simulink model "SwcCanSendFaultV2"  (R2021b)
settings: Solver=ode1  StartTime=0.0  StopTime=15  FixedStep=0.01  RelTol=1e-3
PostLoadFcn:
  | CCM_Parameter
values from neighbouring files (symbols this model uses):
  Fault0x01 = FaultCodeGen(1,timeserise0x01)    [FaultCodeGenerate.m]
  Fault0x02 = FaultCodeGen(2,timeserise0x02)    [FaultCodeGenerate.m]
  Fault0x03 = FaultCodeGen(3,timeserise0x03)    [FaultCodeGenerate.m]
  Fault0x04 = FaultCodeGen(4,timeserise0x04)    [FaultCodeGenerate.m]
  Fault0x05 = FaultCodeGen(5,timeserise0x05)    [FaultCodeGenerate.m]
  Fault0x06 = FaultCodeGen(6,timeserise0x06)    [FaultCodeGenerate.m]
undefined symbols (not defined in the file or in its folder): DiscIntNeverNeededParam
libraries: simulink x2
settings Model: NumberOfSteps=40  Creator=renjianze  LastModifiedBy=renjianze
settings OptimizationCC: DefaultParameterBehavior=Inlined  EnhancedBackFolding=on  PassReuseOutputArgsAs=Individual arguments  ZeroExternalMemoryAtStartup=off  ZeroInternalMemoryAtStartup=off  OptimizeBlockOrder=speed  DifferentSizesBufferReuse=on  OptimizationCustomize=off  EfficientTunableParamExpr=on
settings DebuggingCC: ParameterTunabilityLossMsg=error
settings HardwareCC: ProdBitPerPointer=32  ProdBitPerSizeT=32  ProdBitPerPtrDiffT=32  ProdLargestAtomicInteger=Long  ProdLargestAtomicFloat=Double  ProdWordSize=32  ProdHWDeviceType=NXP->Cortex-M4
settings SFSimCC: MATLABDynamicMemAlloc=off
settings RTWCC: Description=Embedded Coder  SystemTargetFile=ert.tlc  TemplateMakefile=ert_default_tmf  CustomHeaderCode="#include  \"interface.h\""
settings CodeAppCC: ForceParamTrailComments=on  IgnoreCustomStorageClasses=off  OperatorAnnotations=on  SimulinkDataObjDesc=on  SFDataObjDesc=on  InsertBlockDesc=on
settings ERTTargetCC: TargetLangStandard=C99 (ISO)  GenerateSampleERTMain=on  InlinedParameterPlacement=NonHierarchical  ERTCustomFileTemplate=example_file_process.tlc  ERTFilePackagingFormat=Compact

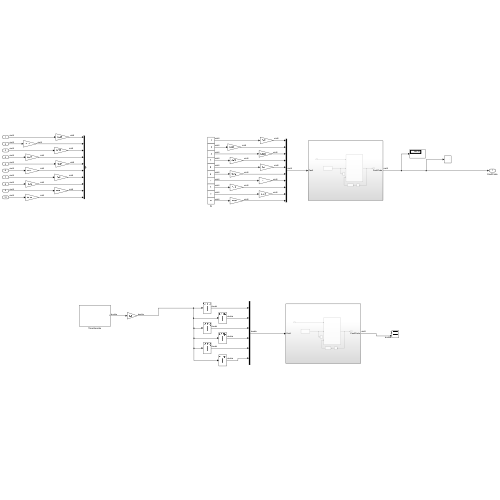
[thumbnail: Simulink's stored preview of the top-level diagram]
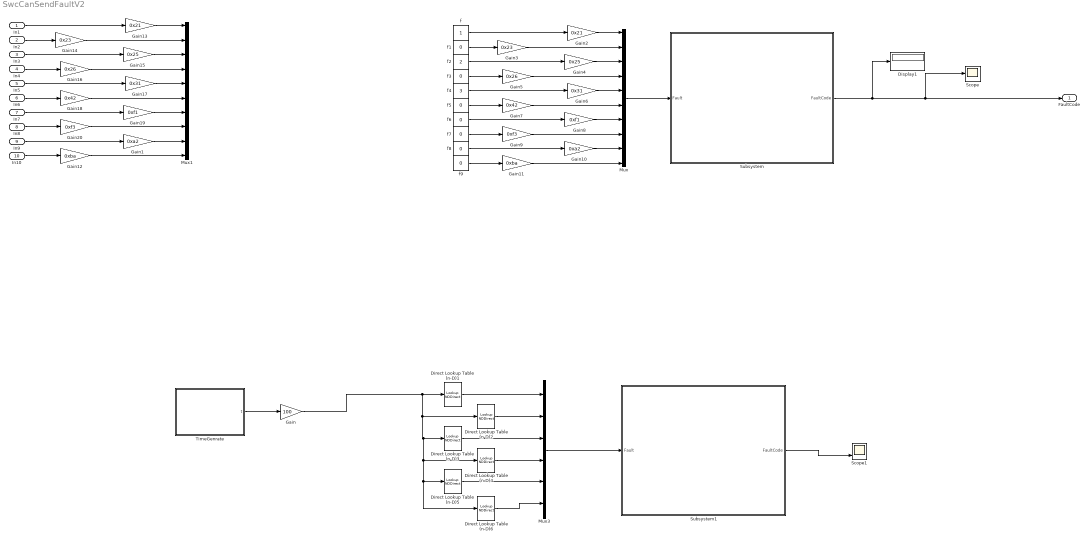
== system SwcCanSendFaultV2 ==
  In1 : Inport
  In2 : Inport  Port=2
  In3 : Inport  Port=3
  In4 : Inport  Port=4
  In5 : Inport  Port=5
  In6 : Inport  Port=6
  In7 : Inport  Port=7
  In8 : Inport  Port=8
  In9 : Inport  Port=9
  In10 : Inport  Port=10
  Direct Lookup Table (n-D)1 : LookupNDDirect  NumberOfTableDimensions=1  Table=Fault0x01
  Direct Lookup Table (n-D)2 : LookupNDDirect  NumberOfTableDimensions=1  Table=Fault0x02
  Direct Lookup Table (n-D)3 : LookupNDDirect  NumberOfTableDimensions=1  Table=Fault0x03
  Direct Lookup Table (n-D)4 : LookupNDDirect  NumberOfTableDimensions=1  Table=Fault0x04
  Direct Lookup Table (n-D)5 : LookupNDDirect  NumberOfTableDimensions=1  Table=Fault0x05
  Direct Lookup Table (n-D)6 : LookupNDDirect  NumberOfTableDimensions=1  Table=Fault0x06
  Display1 : Display
      settings: Format=hex (Stored Integer)
  Gain : Gain  Gain=100
  Gain1 : Gain  Gain=0xa2  ParamDataTypeStr=uint8  OutDataTypeStr=uint8
  Gain10 : Gain  Gain=0xa2  ParamDataTypeStr=uint8  OutDataTypeStr=uint8
  Gain11 : Gain  Gain=0xba  ParamDataTypeStr=uint8  OutDataTypeStr=uint8
  Gain12 : Gain  Gain=0xba  ParamDataTypeStr=uint8  OutDataTypeStr=uint8
  Gain13 : Gain  Gain=0x21  ParamDataTypeStr=uint8  OutDataTypeStr=uint8
  Gain14 : Gain  Gain=0x23  ParamDataTypeStr=uint8  OutDataTypeStr=uint8
  Gain15 : Gain  Gain=0x25  ParamDataTypeStr=uint8  OutDataTypeStr=uint8
  Gain16 : Gain  Gain=0x26  ParamDataTypeStr=uint8  OutDataTypeStr=uint8
  Gain17 : Gain  Gain=0x31  ParamDataTypeStr=uint8  OutDataTypeStr=uint8
  Gain18 : Gain  Gain=0x42  ParamDataTypeStr=uint8  OutDataTypeStr=uint8
  Gain19 : Gain  Gain=0xf1  ParamDataTypeStr=uint8  OutDataTypeStr=uint8
  Gain2 : Gain  Gain=0x21  ParamDataTypeStr=uint8  OutDataTypeStr=uint8
  Gain20 : Gain  Gain=0xf3  ParamDataTypeStr=uint8  OutDataTypeStr=uint8
  Gain3 : Gain  Gain=0x23  ParamDataTypeStr=uint8  OutDataTypeStr=uint8
  Gain4 : Gain  Gain=0x25  ParamDataTypeStr=uint8  OutDataTypeStr=uint8
  Gain5 : Gain  Gain=0x26  ParamDataTypeStr=uint8  OutDataTypeStr=uint8
  Gain6 : Gain  Gain=0x31  ParamDataTypeStr=uint8  OutDataTypeStr=uint8
  Gain7 : Gain  Gain=0x42  ParamDataTypeStr=uint8  OutDataTypeStr=uint8
  Gain8 : Gain  Gain=0xf1  ParamDataTypeStr=uint8  OutDataTypeStr=uint8
  Gain9 : Gain  Gain=0xf3  ParamDataTypeStr=uint8  OutDataTypeStr=uint8
  Mux : Mux  Inputs=[1,1,1,1,1,1,1,1,1,1]
  Mux1 : Mux  Inputs=[1,1,1,1,1,1,1,1,1,1]
  Mux3 : Mux  Inputs=[1,1,1,1,1,1]
  Scope : Scope
  Scope1 : Scope  NumInputPorts=2
  Subsystem : Subsystem
  Subsystem1 : Subsystem
  TimeGenrate : Subsystem
  f : Constant  OutDataTypeStr=uint8
  f{1,3,5..9} (7 alike) : Constant  Value=0  OutDataTypeStr=uint8
  f2 : Constant  Value=2  OutDataTypeStr=uint8
  f4 : Constant  Value=3  OutDataTypeStr=uint8
  FaultCode : Outport
  wires:
  Gain2/1 -> Mux/1
  f/1 -> Gain2/1
  f1/1 -> Gain3/1
  Gain3/1 -> Mux/2
  Gain4/1 -> Mux/3
  f2/1 -> Gain4/1
  f3/1 -> Gain5/1
  Gain5/1 -> Mux/4
  Gain6/1 -> Mux/5
  f4/1 -> Gain6/1
  Gain8/1 -> Mux/7
  f6/1 -> Gain8/1
  f5/1 -> Gain7/1
  Gain7/1 -> Mux/6
  f7/1 -> Gain9/1
  Gain9/1 -> Mux/8
  Gain10/1 -> Mux/9
  f8/1 -> Gain10/1
  f9/1 -> Gain11/1
  Gain11/1 -> Mux/10
  Gain12/1 -> Mux1/10
  In10/1 -> Gain12/1
  Gain19/1 -> Mux1/7
  Gain1/1 -> Mux1/9
  Gain14/1 -> Mux1/2
  Gain17/1 -> Mux1/5
  In1/1 -> Gain13/1
  Gain20/1 -> Mux1/8
  In9/1 -> Gain1/1
  In8/1 -> Gain20/1
  In7/1 -> Gain19/1
  Gain15/1 -> Mux1/3
  In4/1 -> Gain16/1
  In2/1 -> Gain14/1
  In5/1 -> Gain17/1
  Gain18/1 -> Mux1/6
  Gain16/1 -> Mux1/4
  In3/1 -> Gain15/1
  Gain13/1 -> Mux1/1
  In6/1 -> Gain18/1
  Subsystem/1(FaultCode) -> Scope/1, FaultCode/1, Display1/1
  Mux/1 -> Subsystem/1(Fault)
  Mux3/1 -> Subsystem1/1(Fault)
  TimeGenrate/1(t) -> Gain/1
  Gain/1 -> Direct Lookup Table (n-D)2/1, Direct Lookup Table (n-D)6/1, Direct Lookup Table (n-D)5/1, Direct Lookup Table (n-D)4/1, Direct Lookup Table (n-D)3/1, Direct Lookup Table (n-D)1/1
  Direct Lookup Table (n-D)1/1 -> Mux3/1
  Direct Lookup Table (n-D)2/1 -> Mux3/2
  Direct Lookup Table (n-D)3/1 -> Mux3/3
  Direct Lookup Table (n-D)4/1 -> Mux3/4
  Direct Lookup Table (n-D)5/1 -> Mux3/5
  Direct Lookup Table (n-D)6/1 -> Mux3/6
  Subsystem1/1(FaultCode) -> Scope1/2

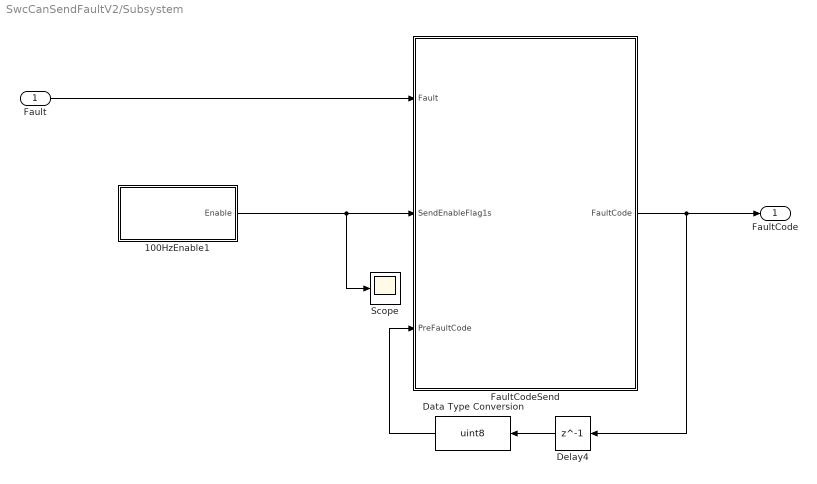
== system SwcCanSendFaultV2/Subsystem ==
  Fault : Inport
  100HzEnable1 : Subsystem  mask{fre=100, EnableTime=1}
      mask prompts: fre "采样频率(Hz)"; EnableTime "使能时间(s)"
  Data Type Conversion : DataTypeConversion  OutDataTypeStr=uint8
  Delay4 : Delay  DelayLength=1
  FaultCodeSend : MATLAB Function  TreatAsAtomicUnit=on
  Scope : Scope
  FaultCode : Outport
  wires:
  100HzEnable1/1(Enable) -> FaultCodeSend/2(SendEnableFlag1s), Scope/1
  Delay4/1 -> Data Type Conversion/1
  FaultCodeSend/1(FaultCode) -> Delay4/1, FaultCode/1
  Fault/1 -> FaultCodeSend/1(Fault)
  Data Type Conversion/1 -> FaultCodeSend/3(PreFaultCode)

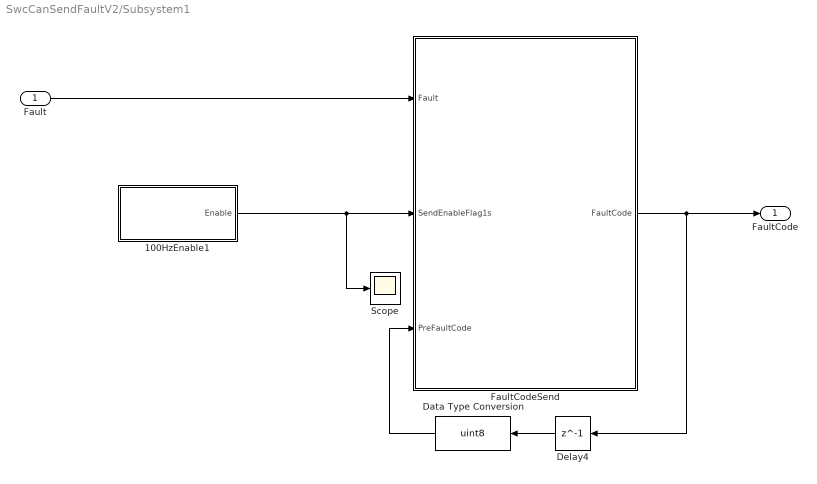
== system SwcCanSendFaultV2/Subsystem1 ==
  Fault : Inport
  100HzEnable1 : Subsystem  mask{fre=100, EnableTime=1}
      mask prompts: fre "采样频率(Hz)"; EnableTime "使能时间(s)"
  Data Type Conversion : DataTypeConversion  OutDataTypeStr=uint8
  Delay4 : Delay  DelayLength=1
  FaultCodeSend : MATLAB Function  TreatAsAtomicUnit=on
  Scope : Scope
  FaultCode : Outport
  wires:
  100HzEnable1/1(Enable) -> FaultCodeSend/2(SendEnableFlag1s), Scope/1
  Delay4/1 -> Data Type Conversion/1
  FaultCodeSend/1(FaultCode) -> Delay4/1, FaultCode/1
  Fault/1 -> FaultCodeSend/1(Fault)
  Data Type Conversion/1 -> FaultCodeSend/3(PreFaultCode)

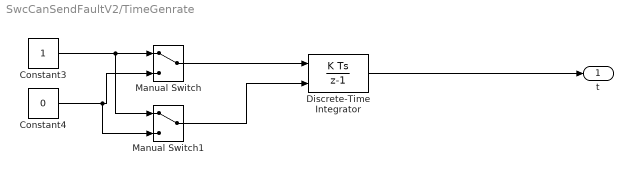
== system SwcCanSendFaultV2/TimeGenrate ==
  Constant3 : Constant
  Constant4 : Constant  Value=0
  Discrete-Time Integrator : DiscreteIntegrator  ExternalReset=either  SampleTime=-1  ICPrevOutput=DiscIntNeverNeededParam  ICPrevScaledInput=DiscIntNeverNeededParam
  Manual Switch : ManualSwitch
  Manual Switch1 : ManualSwitch
  t : Outport
  wires:
  Constant3/1 -> Manual Switch1/1, Manual Switch/1
  Constant4/1 -> Manual Switch1/2, Manual Switch/2
  Manual Switch1/1 -> Discrete-Time Integrator/2
  Discrete-Time Integrator/1 -> t/1
  Manual Switch/1 -> Discrete-Time Integrator/1

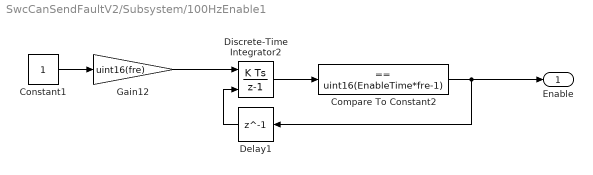
== system SwcCanSendFaultV2/Subsystem/100HzEnable1 ==
  Compare To Constant2 : simulink/Logic and Bit Operations/Compare To Constant  relop===  const=uint16(EnableTime*fre-1)  OutDataTypeStr=boolean
  Constant1 : Constant
  Delay1 : Delay  DelayLength=1
  Discrete-Time Integrator2 : DiscreteIntegrator  ExternalReset=rising  SampleTime=-1  ICPrevOutput=DiscIntNeverNeededParam  ICPrevScaledInput=DiscIntNeverNeededParam
  Gain12 : Gain  Gain=uint16(fre)
  Enable : Outport
  wires:
  Delay1/1 -> Discrete-Time Integrator2/2
  Compare To Constant2/1 -> Delay1/1, Enable/1
  Discrete-Time Integrator2/1 -> Compare To Constant2/1
  Constant1/1 -> Gain12/1
  Gain12/1 -> Discrete-Time Integrator2/1

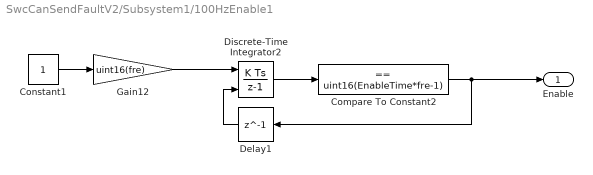
== system SwcCanSendFaultV2/Subsystem1/100HzEnable1 ==
  Compare To Constant2 : simulink/Logic and Bit Operations/Compare To Constant  relop===  const=uint16(EnableTime*fre-1)  OutDataTypeStr=boolean
  Constant1 : Constant
  Delay1 : Delay  DelayLength=1
  Discrete-Time Integrator2 : DiscreteIntegrator  ExternalReset=rising  SampleTime=-1  ICPrevOutput=DiscIntNeverNeededParam  ICPrevScaledInput=DiscIntNeverNeededParam
  Gain12 : Gain  Gain=uint16(fre)
  Enable : Outport
  wires:
  Delay1/1 -> Discrete-Time Integrator2/2
  Compare To Constant2/1 -> Delay1/1, Enable/1
  Discrete-Time Integrator2/1 -> Compare To Constant2/1
  Constant1/1 -> Gain12/1
  Gain12/1 -> Discrete-Time Integrator2/1

== matlab function SwcCanSendFaultV2/Subsystem1/FaultCodeSend ==
  data: Fault input; FaultCode output; SendEnableFlag1s input; PreFaultCode input
function FaultCode = fcn(Fault,SendEnableFlag1s,PreFaultCode)

%% 赋初值
persistent Temp               %% 错误缓存区
persistent cannum             %% 错误发送位
persistent WriteEnableFlag    %% 清除错误码

    if isempty(cannum)
        cannum = 0;
    end

    if isempty(WriteEnableFlag)
        WriteEnableFlag = zeros(length(Fault),1);
    end

%% 更新缓存区
     if isempty(Temp)
         Temp = Fault; % 
     else
       for i = 1:length(Fault)
           if Fault(i) > Temp(i)    %假设错误只有1和0
               Temp(i) = Fault(i);
           elseif   WriteEnableFlag(i) == 1
               Temp(i) = Fault(i);
               WriteEnableFlag(i) =0;
           end
       end
     end
  
%% 确认发送的错误
if SendEnableFlag1s == 1
    if all(Temp == 0)
            FaultCode = uint8(0);
    else
            for i = 1:length(Temp)
                %=============================
                    cannum = cannum + 1;
                    if cannum > length(Temp)
                        cannum = 1;
                    end
                    if Temp(cannum) ~= 0
                        FaultCode = uint8(Temp(cannum));
                        WriteEnableFlag(cannum) = 1;
                        break
                    else               
                        FaultCode = uint8(0);
                    end
            end 
                %=============================
    end
else
    FaultCode = uint8(PreFaultCode);
end
validateattributes(FaultCode, {'uint8'}, {}); 

end

== matlab function SwcCanSendFaultV2/Subsystem/FaultCodeSend ==
  data: Fault input; FaultCode output; SendEnableFlag1s input; PreFaultCode input
function FaultCode = fcn(Fault,SendEnableFlag1s,PreFaultCode)

%% 赋初值
persistent Temp               %% 错误缓存区
persistent cannum             %% 错误发送位
persistent WriteEnableFlag    %% 清除错误码

    if isempty(cannum)
        cannum = 0;
    end

    if isempty(WriteEnableFlag)
        WriteEnableFlag = zeros(length(Fault),1);
    end

%% 更新缓存区
     if isempty(Temp)
         Temp = Fault; % 
     else
       for i = 1:length(Fault)
           if Fault(i) > Temp(i)    %假设错误只有1和0
               Temp(i) = Fault(i);
           elseif   WriteEnableFlag(i) == 1
               Temp(i) = Fault(i);
               WriteEnableFlag(i) =0;
           end
       end
     end
  
%% 确认发送的错误
if SendEnableFlag1s == 1
    if all(Temp == 0)
            FaultCode = uint8(0);
    else
            for i = 1:length(Temp)
                %=============================
                    cannum = cannum + 1;
                    if cannum > length(Temp)
                        cannum = 1;
                    end
                    if Temp(cannum) ~= 0
                        FaultCode = uint8(Temp(cannum));
                        WriteEnableFlag(cannum) = 1;
                        break
                    else               
                        FaultCode = uint8(0);
                    end
            end 
                %=============================
    end
else
    FaultCode = uint8(PreFaultCode);
end
validateattributes(FaultCode, {'uint8'}, {}); 

end
